simulink model "sineWaveTest"  (R2023b)
settings: Solver=VariableStepAuto  StartTime=0.0  StopTime=15  MaxStep=0.001  RelTol=1e-3
libraries: SignalEditorBlockLib x2
settings Model: Creator=grouleau  LastModifiedBy=grouleau

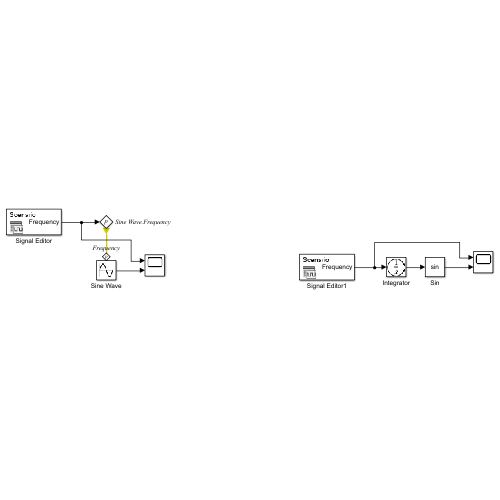
[thumbnail: Simulink's stored preview of the top-level diagram]
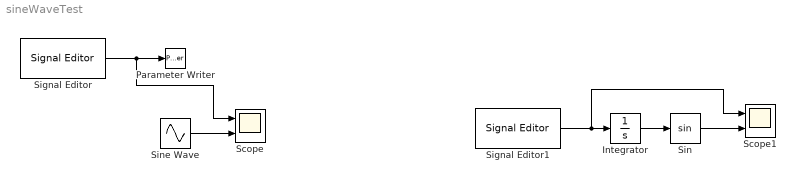
== system sineWaveTest ==
  Integrator : Integrator  WrapState=on  WrappedStateUpperValue=2*pi  WrappedStateLowerValue=0
  Parameter Writer : ParameterWriter  ParameterOwnerBlock=../Sine Wave  ParameterName=Frequency  ParameterInternalName=Frequency
  Scope : Scope  NumInputPorts=2
  Scope1 : Scope  NumInputPorts=2
  Signal Editor : SignalEditorBlockLib/Signal Editor  FileName=FrequencyRamp.mat  ActiveScenario=Scenario  ActiveSignal=Frequency  IsBus=off  OutputBusObjectStr=Bus: BusObject  SampleTime=0  ZeroCross=off  OutputAfterFinalValue=Setting to zero  Unit=inherit  PreserveSignalName=on  ApplySigPropsToAllScenarios=on  ApplySigPropsToAllSignals=off
  Signal Editor1 : SignalEditorBlockLib/Signal Editor  FileName=FrequencyRamp.mat  ActiveScenario=Scenario  ActiveSignal=Frequency  IsBus=off  OutputBusObjectStr=Bus: BusObject  SampleTime=0  ZeroCross=off  OutputAfterFinalValue=Setting to zero  Unit=inherit  PreserveSignalName=on  ApplySigPropsToAllScenarios=on  ApplySigPropsToAllSignals=off
  Sin : Trigonometry
  Sine Wave : Sin  SampleTime=0
  wires:
  Sine Wave/1 -> Scope/2
  Signal Editor/1 -> Scope/1, Parameter Writer/1
  Sin/1 -> Scope1/2
  Integrator/1 -> Sin/1
  Signal Editor1/1 -> Scope1/1, Integrator/1
